simulink model "simulacion"  (R2019b)
settings: Solver=ode4  StartTime=0.0  StopTime=10  FixedStep=10e-6  RelTol=1e-3
libraries: cstblocks x4
settings Model: Creator=mpier  LastModifiedBy=rochi

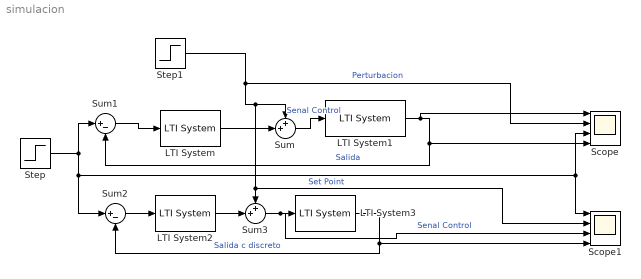
== system simulacion ==
  LTI System : cstblocks/LTI System  sys=c  IC=[]
  LTI System1 : cstblocks/LTI System  sys=planta  IC=[]
  LTI System2 : cstblocks/LTI System  sys=c_disc  IC=[]
  LTI System3 : cstblocks/LTI System  sys=planta_disc  IC=[]
  Scope : Scope  NumInputPorts=4
  Scope1 : Scope  NumInputPorts=4
  Step : Step  SampleTime=0
  Step1 : Step  Time=5  After=10  SampleTime=0
  Sum : Sum  Inputs=++|
  Sum1 : Sum  Inputs=|+-
  Sum2 : Sum  Inputs=|+-
  Sum3 : Sum  Inputs=++|
  wires:
  LTI System/1 -> Sum/2
  Sum/1 -> LTI System1/1  "Senal Control"
  Sum1/1 -> LTI System/1
  LTI System1/1 -> Scope/1, Scope/4, Sum1/2  "Salida"
  Step/1 -> Scope1/1, Scope/3, Sum2/1, Sum1/1  "Set Point"
  Step1/1 -> Scope/2, Scope1/2, Sum3/1, Sum/1  "Perturbacion"
  Sum2/1 -> LTI System2/1
  LTI System3/1 -> Scope1/4, Sum2/2  "Salida c discreto"
  LTI System2/1 -> Sum3/2
  Sum3/1 -> Scope1/3, LTI System3/1  "Senal Control"
